simulink library "SUB_ECU_L4_MABX_HW_Interface"  (R2018a)
settings: Solver=VariableStepAuto  StartTime=0.0  StopTime=10.0  RelTol=1e-3
PostLoadFcn:
  | , if any(exist('dsrtsu_mdlpostloadfcn', 'file') == [2, 3, 6]), try dsrtsu_mdlpostloadfcn('Execute', bdroot); catch fprintf('Error in PostLoadFcn (dsrtsu_mdlpostloadfcn) for model "%s":\n %s\n', bdroot, lasterr); end, end,
undefined symbols (not defined in the file or in its folder): CANR_PROPB_REAX_3_13_CHANNEL_APV, CANR_PROPB_REAX_4_13_CHANNEL_APV, CANR_PROPB_XPR_1_50_CHANNEL_APV, ENUM_CAN_RX_T, ENUM_CAN_TX_T, ENUM_REAX_OPERATION_MODE_T, ENUM_SIGNAL_HEALTH_T, ENUM_XBR_CONTROL_MODE_T, ENUM_XBR_EBI_MODE_T, ENUM_XBR_PASS_THROUGH_ACTIVE_T, ENUM_XBR_PRIORITY_T, ENUM_XPR_INHIBIT_PARK_MANUAL_T, ENUM_XPR_INHIBIT_UNPARK_MANUAL_T, ENUM_XPR_PARK_MANUAL_T, ENUM_XPR_UNPARK_MANUAL_T, PROPB_REAX_1_E4_DES_POS_SIG_SRC_APV, PROPB_REAX_1_E4_DESIRED_OPMODE_APV, PROPB_REAX_1_E4_DESIRED_POSITION_APV, ptc_matlab_lib
libraries: PTC_MBDS_LIB x264, rtican x172, EmE_MBD_Blockset x39, simulink x34, $bdroot x16, rti1401lib_dio_type4 x8, simulink_need_slupdate x7, dsa_tcpip_lib x4, rti1401lib_adc_type4 x3, rtmapslib x3, rtitasklib x3
(part 48 of 51)

== system SUB_ECU_L4_MABX_HW_Interface/CAN_Out_PTC_1571/CAN_TX_100ms/Encode_PropB_XPR_FC/Encode_PropB_XPR_FC_checksum ==
  byte1 : Inport  OutDataTypeStr=uint8
  byte2 : Inport  Port=2  OutDataTypeStr=uint8
  byte3 : Inport  Port=3
  byte4 : Inport  Port=4
  byte5 : Inport  Port=5
  byte6 : Inport  Port=6
  byte7 : Inport  Port=7
  Counter : Inport  Port=8
  MessageID : Inport  Port=9
  AND1 : PTC_MBDS_LIB/MBDS Standard Library/Basic Operations/Logic and Bit Operations/AND  BitwiseMode=on  Inputs=1  UseBitMask=on  BitMask='0F'  OutDataTypeStr=uint8  PTC_MBDS_BlockVersion=5.41  PTC_BlockType=PTC_MBDS_AND
      settings: AttributesFormatString=bitwise  SourceProductName=PACCAR Technical Center MBDS Library
  AND10 : PTC_MBDS_LIB/MBDS Standard Library/Basic Operations/Logic and Bit Operations/AND  BitwiseMode=on  Inputs=1  UseBitMask=on  BitMask='0F'  OutDataTypeStr=uint8  PTC_MBDS_BlockVersion=5.41  PTC_BlockType=PTC_MBDS_AND
      settings: AttributesFormatString=bitwise  SourceProductName=PACCAR Technical Center MBDS Library
  AND5 : PTC_MBDS_LIB/MBDS Standard Library/Basic Operations/Logic and Bit Operations/AND  BitwiseMode=on  Inputs=1  UseBitMask=on  BitMask='000000FF'  OutDataTypeStr=uint8  PTC_MBDS_BlockVersion=5.41  PTC_BlockType=PTC_MBDS_AND
      settings: AttributesFormatString=bitwise  SourceProductName=PACCAR Technical Center MBDS Library
  AND6 : PTC_MBDS_LIB/MBDS Standard Library/Basic Operations/Logic and Bit Operations/AND  BitwiseMode=on  Inputs=1  UseBitMask=on  BitMask='0000FF00'  OutDataTypeStr=uint16  PTC_MBDS_BlockVersion=5.41  PTC_BlockType=PTC_MBDS_AND
      settings: AttributesFormatString=bitwise  SourceProductName=PACCAR Technical Center MBDS Library
  AND7 : PTC_MBDS_LIB/MBDS Standard Library/Basic Operations/Logic and Bit Operations/AND  BitwiseMode=on  Inputs=1  UseBitMask=on  BitMask='00FF0000'  OutDataTypeStr=uint32  PTC_MBDS_BlockVersion=5.41  PTC_BlockType=PTC_MBDS_AND
      settings: AttributesFormatString=bitwise  SourceProductName=PACCAR Technical Center MBDS Library
  AND8 : PTC_MBDS_LIB/MBDS Standard Library/Basic Operations/Logic and Bit Operations/AND  BitwiseMode=on  Inputs=1  UseBitMask=on  BitMask='FF000000'  OutDataTypeStr=uint32  PTC_MBDS_BlockVersion=5.41  PTC_BlockType=PTC_MBDS_AND
      settings: AttributesFormatString=bitwise  SourceProductName=PACCAR Technical Center MBDS Library
  Add : Sum  Inputs=++++++++++++  OutDataTypeStr=uint8  InputSameDT=on
      settings: AttributesFormatString=Saturate: %<SaturateOnIntegerOverflow>
  Add1 : Sum  OutDataTypeStr=uint8  InputSameDT=on
      settings: AttributesFormatString=Saturate: %<SaturateOnIntegerOverflow>
  Data Type Conversion10 : DataTypeConversion  OutDataTypeStr=uint8  SaturateOnIntegerOverflow=on
  Data Type Conversion11 : DataTypeConversion  OutDataTypeStr=uint8  SaturateOnIntegerOverflow=on
  Data Type Conversion13 : DataTypeConversion  OutMin=0  OutMax=15  OutDataTypeStr=uint8  SaturateOnIntegerOverflow=on
  Data Type Conversion8 : DataTypeConversion  OutDataTypeStr=uint32  SaturateOnIntegerOverflow=on
  Data Type Conversion9 : DataTypeConversion  OutDataTypeStr=uint8  SaturateOnIntegerOverflow=on
  Shift_Arithmetic 3 : ArithShift  BitShiftNumber=8
  Shift_Arithmetic 4 : ArithShift  BitShiftNumber=16
  Shift_Arithmetic 5 : ArithShift  BitShiftNumber=24
  Shift_Arithmetic 7 : ArithShift  BitShiftNumber=4
  Data : Outport
  wires:
  MessageID/1 -> Data Type Conversion8/1
  Data Type Conversion8/1 -> AND8/1, AND7/1, AND6/1, AND5/1
  AND5/1 -> Add/8  "MessageIDLowByte"
  AND6/1 -> Shift_Arithmetic 3/1
  Shift_Arithmetic 3/1 -> Data Type Conversion9/1
  Data Type Conversion9/1 -> Add/9  "MessageIDMidLowByte"
  AND7/1 -> Shift_Arithmetic 4/1
  Shift_Arithmetic 4/1 -> Data Type Conversion10/1
  Data Type Conversion10/1 -> Add/10  "MessageIDMidHighByte"
  AND8/1 -> Shift_Arithmetic 5/1
  Shift_Arithmetic 5/1 -> Data Type Conversion11/1
  Data Type Conversion11/1 -> Add/11  "MessageIDHighByte"
  AND10/1 -> Add/12
  AND1/1 -> Data/1
  Counter/1 -> Data Type Conversion13/1
  Data Type Conversion13/1 -> AND10/1
  byte1/1 -> Add/1
  byte2/1 -> Add/2
  byte3/1 -> Add/3
  byte4/1 -> Add/4
  byte5/1 -> Add/5
  byte6/1 -> Add/6
  byte7/1 -> Add/7
  Add/1 -> Add1/2, Shift_Arithmetic 7/1  "Checksum"
  Shift_Arithmetic 7/1 -> Add1/1
  Add1/1 -> AND1/1

== system SUB_ECU_L4_MABX_HW_Interface/CAN_Out_PTC_1571/CAN_TX_100ms/Encode_PropB_XPR_FC/MessageID ==
  note: 0x18FF04FC
  Data Type Conversion{,1..5} (6 alike) : DataTypeConversion  OutDataTypeStr=uint32  SaturateOnIntegerOverflow=on
  DataPage : Constant  Value=boolean(0)
  ExtendedDataPage : Constant  Value=boolean(0)
  OR : PTC_MBDS_LIB/MBDS Standard Library/Basic Operations/Logic and Bit Operations/OR  BitwiseMode=on  Inputs=6  UseBitMask=off  BitMask='A7'  OutDataTypeStr=Inherit: Inherit via back propagation  PTC_MBDS_BlockVersion=5.41  PTC_BlockType=PTC_MBDS_OR
      settings: AttributesFormatString=bitwise  SourceProductName=PACCAR Technical Center MBDS Library
  PDUFormat : Constant  Value=uint8(hex2dec('FF'))
  PDUSpecific : Constant  Value=uint8(hex2dec('04'))
  Priority : Constant  Value=uint8(6)
  "Shift_Arithmetic " : ArithShift  BitShiftNumber=-26
  Shift_Arithmetic 1 : ArithShift  BitShiftNumber=-25
  Shift_Arithmetic 2 : ArithShift  BitShiftNumber=-24
  Shift_Arithmetic 3 : ArithShift  BitShiftNumber=-16
  Shift_Arithmetic 4 : ArithShift  BitShiftNumber=-8
  SourceAddress : Constant  Value=uint8(hex2dec('FC'))
  MessageID : Outport
  wires:
  Shift_Arithmetic 3/1 -> OR/4
  Shift_Arithmetic 4/1 -> OR/5
  Shift_Arithmetic 2/1 -> OR/3
  Shift_Arithmetic 1/1 -> OR/2
  "Shift_Arithmetic "/1 -> OR/1
  Data Type Conversion5/1 -> OR/6
  SourceAddress/1 -> Data Type Conversion5/1
  Data Type Conversion4/1 -> Shift_Arithmetic 4/1
  PDUSpecific/1 -> Data Type Conversion4/1
  Data Type Conversion3/1 -> Shift_Arithmetic 3/1
  PDUFormat/1 -> Data Type Conversion3/1
  Data Type Conversion2/1 -> Shift_Arithmetic 2/1
  DataPage/1 -> Data Type Conversion2/1
  Data Type Conversion1/1 -> Shift_Arithmetic 1/1
  ExtendedDataPage/1 -> Data Type Conversion1/1
  Data Type Conversion/1 -> "Shift_Arithmetic "/1
  Priority/1 -> Data Type Conversion/1
  OR/1 -> MessageID/1

== system SUB_ECU_L4_MABX_HW_Interface/CAN_Out_PTC_1571/CAN_TX_100ms/Encode_PropB_XPR_FC/Rolling_15_counter ==
  Enable : EnablePort  ZeroCross=off
      settings: AttributesFormatString=States when enabling: %<StatesWhenEnabling>
  Increment Real World1 : simulink/Additional Math & Discrete/Additional Math: Increment - Decrement/Increment Real World  DisableCoverage=on
      settings: SourceProductName=Simulink  SourceProductBaseCode=SL
  Unit_Delay : UnitDelay  SampleTime=-1
      settings: AttributesFormatString=IC: %<vinit>
  Wrap To Zero1 : simulink/Discontinuities/Wrap To Zero  DisableCoverage=on  Threshold=15
      settings: SourceProductName=Simulink  SourceProductBaseCode=SL
  Rolling_15_counter : Outport  InitialOutput=15
      settings: AttributesFormatString=IC: %<InitialOutput>\nDisabled Value: %<OutputWhenDisabled>\n
  wires:
  Unit_Delay/1 -> Rolling_15_counter/1, Increment Real World1/1
  Wrap To Zero1/1 -> Unit_Delay/1
  Increment Real World1/1 -> Wrap To Zero1/1

== system SUB_ECU_L4_MABX_HW_Interface/CAN_Out_PTC_1571/CAN_TX_100ms/POSRapidUpdate/TX ==
  Enable : Inport
  Data : Inport  Port=2
  Bus Selector : BusSelector  OutputSignals=INPUTS.CAN.PosRapidUpdate.Latitude_,INPUTS.CAN.PosRapidUpdate.Longitude_
  Data Type Conversion : DataTypeConversion  OutDataTypeStr=double
  Data Type Conversion1 : DataTypeConversion  OutDataTypeStr=double
  Std_PosRapidUpdate_01 : rtican/RTICAN Transmit (TX)   Reserved1=[]  Reserved2=[]  Reserved3=[]  Reserved4=[]  SfcnMessage=[]  Msg_Struct=[]  BoardTypeNo=[]  BoardNo=[]  ChannelNo=[]  Parameters=[]  DialogFcn=[]  UnitName=[]  Revision=[]  UnitValues=[]  DSProperties=struct('RTI',struct('Version',uint32(5),'BlockType',struct('isSLSource',uint8(1),'isSLSink',uint8(1),'isHWSource',uint8(0),'isHWSink',uint8(0),'isSetup',uint8(0),'isInline',uint8(1),'isNonInline',uint8(0),'isInterrupt',uint8(0),'isChannelwise',uint8(0)),'IOBoardType','RTICAN','UnitType','MESSAGE','Identifier','TX','DialogType','MSVC','BlockSet','RTICAN','SlaveProcessor','CAN'))  RTIBlockInterface=struct('InputPortsWidth',int32([1 1]),'InputPortsActive',[1 1],'InputPortsName',{{'Latitude_','Longitude_'}},'InputPortsDataType',{{'SS_DOUBLE','SS_DOUBLE'}},'OutputPortsWidth',int32([1 1 1 1]),'OutputPortsActive',[1 1 1 1],'OutputPortsName',{{['TX status'],['TX time'],['TX delta time'],['TX delay time']}},'DialogFcn','rtican_message_interface_gui','BlockDisplay',{{'','center'}},'IconTransparency','on','InitLevel',3,'BlockName',struct('Token',{{'Std_PosRapidUpdate_01'}}),'SampleTime',{{-1}},'TriggerPort',{{'none'}},'EnablePort',{{'yes'}})  RTIBlockParameters=struct('BoardTypeNo',{{1,'OFF',[]}},'BoardNo',{{3,'ON',[1 16]}},'ChannelNo',{{2,'ON',[1 2]}},'Parameters',{{struct('DataFileSupport',struct('DataFileSelectedMaster',1,'DataFileSelectedLocal',0,'DataFileName','c:\data\svn\truck1571\dbc\mabx_can6.dbc|c:\data\svn\candb\mabx_can4_chrisbalton.dbc|','DataFileDate',{{{['12-Oct-2017 12:26:19']},{''}}},'SelectedFile',['<no file selected>']),'Options',struct('StatusSelected',1,'TimeSelected',1,'DeltaTimeSelected',1,'DelayTimeSelected',1,'DelayTimeTXCommandSelected',0,'EncodeSetUnusedBitsToOne',1,'EnableMsgLoopback',0,'TriggerPort',struct('Selected',0,'TriggerType',0),'EnablePortSelected',1,'SignalOnPortnameSelected',1,'UserCoding',struct('Selected',0,'InterfaceFile','UserEncodingFile','FcnName','UserEncodeFcn','InportSelected',0,'InportWidth',1,'OutportSelected',0,'OutportWidth',1),'TerminationMsg',struct('Selected',0,'Byte0_7','0'),'InitialMsg',struct('Selected',0,'Byte0_7','0')),'Message',struct('MsgOnBlocknameSelected',1,'MsgName','Std_PosRapidUpdate_01','MsgIdFormat',0,'MsgId',3,'MsgLength',8,'NumSignals',2,'SampleTime',-1,'StartTime',struct('Selected',0,'Value',0),'AutoRepeatTime',struct('Selected',0,'Value',0.1),'Timeout',struct('Selected',0,'Value',0.1),'DelayTime',struct('Selected',0,'Value',0.1),'Signal',struct('SgnName',{'Latitude_','Longitude_'},'SgnStartBit',{0,32},'SgnLength',{32,32},'SgnType',{0,0},'ModeValue',{-1,-1},'DataType',{1,1},'ByteLayout',{0,0},'Factor',{1e-7,1e-7},'Offset',{0,0},'SgnComment',{{''},{''}},'SgnUnit',{'deg','deg'},'Min',{-90,-180},'Max',{90,180},'SLDataType',{'SS_DOUBLE','SS_DOUBLE'}),'MsgIdNumFormat',0,'MsgComment',{{['This PGN provides latitude and longitude referenced to WGS84.Being defined as single frame Msg,as ']}}),'Version',1.2,'general',struct('isFromLib',0)),'OFF',[]}},'GroupId',{{struct('Group',{{'RTICAN'}},'No',6,'Behavior',{{'NAMECHANGE'}},'BlockType',{{'SINK'}},'NameChangeFlag',0),'OFF',[]}},'SFcnRTICANMessage',{{struct('MsgType','TX','SFcnPortType','Scalar','MsgName','Std_PosRapidUpdate_01','MsgIdFormat','STD','MsgId',3,'MsgLength',8,'NumSignals',2,'SampleTime',-1,'StartTime',struct('Selected','no','Value',0),'AutoRepeatTime',struct('Selected','no','Value',0.1),'Timeout',struct('Selected','no','Value',0.1),'Signal',struct('SgnName',{'Latitude_','Longitude_'},'SgnStartBit',{0,32},'SgnLength',{32,32},'SgnType',{'standard','standard'},'ModeValue',{-1,-1},'DataType',{['signed int'],['signed int']},'ByteLayout',{['little endian'],['little endian']},'Factor',{1e-7,1e-7},'Offset',{0,0},'SLDataType',{'SS_DOUBLE','SS_DOUBLE'}),'StatusSelected','yes','TimeSelected','yes','DeltaTimeSelected','yes','DelayTimeSelected','yes','DelayTimeTXCommandSelected','no','EncodeSetUnusedBitsToOne','yes','EnableMsgLoopback','no','TriggerPort',struct('Selected','no','TriggerType',0),'EnablePortSelected','yes','UserCoding',struct('Selected','no','InterfaceFile','UserEncodingFile','FcnName','UserEncodeFcn','InportSelected','no','InportWidth',1,'OutportSelected','no','OutportWidth',1),'TerminationMsg',struct('Selected','no','Byte0','0x00','Byte1','0x00','Byte2','0x00','Byte3','0x00','Byte4','0x00','Byte5','0x00','Byte6','0x00','Byte7','0x00'),'InitialMsg',struct('Selected','no','Byte0','0x00','Byte1','0x00','Byte2','0x00','Byte3','0x00','Byte4','0x00','Byte5','0x00','Byte6','0x00','Byte7','0x00'),'BoardType','DS1','BoardNo',3,'ControllerNo',2),'OFF',[]}},'TLCFileName',{{'rtican_tx_message','OFF',[]}})  RTISFcnParameters=struct('SFcnRTICANMessage','struct','TLCFileName','char')  RTIBlockParaDefault=struct('BoardTypeNo',4302,'BoardNo',1,'ChannelNo',1,'Parameters',struct('DataFileSupport',struct('DataFileSelectedMaster',0,'DataFileSelectedLocal',0,'DataFileName','','DataFileDate','','SelectedFile',['<no file selected>']),'Options',struct('StatusSelected',1,'TimeSelected',1,'DeltaTimeSelected',1,'DelayTimeSelected',1,'DelayTimeTXCommandSelected',0,'EncodeSetUnusedBitsToOne',0,'EnableMsgLoopback',0,'TriggerPort',struct('Selected',0,'TriggerType','rising'),'EnablePortSelected',0,'SignalOnPortnameSelected',1,'UserCoding',struct('Selected',0,'InterfaceFile','UserEncodingFile','FcnName','UserEncodeFcn','InportSelected',0,'InportWidth',1,'OutportSelected',0,'OutportWidth',1),'TerminationMsg',struct('Selected',0,'Byte0_7','0'),'InitialMsg',struct('Selected',0,'Byte0_7','0')),'Message',struct('MsgOnBlocknameSelected',0,'MsgName',['TX Message'],'MsgIdFormat',0,'MsgId',100,'MsgLength',8,'NumSignals',1,'SampleTime',-1,'StartTime',struct('Selected',0,'Value',0),'AutoRepeatTime',struct('Selected',0,'Value',0.1),'Timeout',struct('Selected',0,'Value',0.1),'DelayTime',struct('Selected',0,'Value',0.1),'Signal',struct('SgnName',['TX signal'],'SgnStartBit',0,'SgnLength',8,'SgnType',0,'ModeValue',-1,'DataType',0,'SLDataType','SS_DOUBLE','ByteLayout',0,'Factor',1,'Offset',0,'Min',0,'Max',255,'SgnComment',{{}},'SgnUnit',''),'MsgIdNumFormat',0,'MsgComment',{{''}}),'Version',1.2,'general',struct('isFromLib',1)),'GroupId',struct('Group',{{'RTICAN'}},'No',1,'Behavior',{{'NAMECHANGE'}},'BlockType',{{'SINK'}},'NameChangeFlag',0),'SFcnRTICANMessage',struct('MsgType','TX','MsgName',['TX Message'],'MsgIdFormat','STD','MsgId',100,'MsgLength',2,'NumSignals',1,'SampleTime',-1,'StartTime',struct('Selected','no','Value',0),'AutoRepeatTime',struct('Selected','no','Value',0.1),'Timeout',struct('Selected','no','Value',0.1),'DelayTime',struct('Selected','no','Value',0.1),'Signal',struct('SgnName',['TX signal'],'SgnStartBit',0,'SgnLength',8,'SgnType','standard','ModeValue',-1,'DataType',['unsigned int'],'ByteLayout',['little endian'],'SLDataType','SS_DOUBLE','Factor',1,'Offset',0),'StatusSelected','yes','TimeSelected','yes','DeltaTimeSelected','yes','DelayTimeSelected','yes','EnablePortSelected','no','EnableMsgLoopback','no','DelayTimeTXCommandSelected','no','EncodeSetUnusedBitsToOne','no','UserCoding',struct('Selected','no','InterfaceFile','UserDecodingFile','FcnName','UserDecodeFcn','InportSelected','no','InportWidth',1,'OutportSelected','no','OutportWidth',1),'TerminationMsg',struct('Selected','no','Byte0','0x00','Byte1','0x00','Byte2','0x00','Byte3','0x00','Byte4','0x00','Byte5','0x00','Byte6','0x00','Byte7','0x00'),'InitialMsg',struct('Selected','no','Byte0','0x00','Byte1','0x00','Byte2','0x00','Byte3','0x00','Byte4','0x00','Byte5','0x00','Byte6','0x00','Byte7','0x00'),'TriggerPort',struct('Selected','no','TriggerType','rising'),'BoardType','DS4302','BoardNo',1,'ControllerNo',1,'SFcnPortType','Scalar'),'TLCFileName','rtican_tx_message')
      settings: AttributesFormatString=Group Id: RTICAN6\n  SourceProductName=dSPACE RTI CAN Blockset
  Terminator{,1..3} (4 alike) : Terminator
      settings: InitFcn=|
      | try
      |    MBDS_BlockCallback('Update', gcb);
      | end
  wires:
  Data Type Conversion1/1 -> Std_PosRapidUpdate_01/2
  Data Type Conversion/1 -> Std_PosRapidUpdate_01/1
  Enable/1 -> Std_PosRapidUpdate_01/Enable
  Std_PosRapidUpdate_01/2 -> Terminator1/1
  Std_PosRapidUpdate_01/4 -> Terminator3/1
  Std_PosRapidUpdate_01/3 -> Terminator2/1
  Std_PosRapidUpdate_01/1 -> Terminator/1
  Data/1 -> Bus Selector/1
  Bus Selector/1 -> Data Type Conversion/1  "<Latitude_>"
  Bus Selector/2 -> Data Type Conversion1/1  "<Longitude_>"

== system SUB_ECU_L4_MABX_HW_Interface/CAN_Out_PTC_1571/CAN_TX_10ms/CAN_TX_ACCS_E4/TX_CAN4 ==
  note: THIS MESSAGE EXISTS FOR CANALYZER DEBUGGING PURPOSES
      | ONLY AND HAS NO CONTROLLERS EXPECTING TO RECEIVE IT ON ANY CAN BUS
  Enable : Inport
  Data : Inport  Port=2
  ACCS : rtican/RTICAN Transmit (TX)   Reserved1=[]  Reserved2=[]  Reserved3=[]  Reserved4=[]  SfcnMessage=[]  Msg_Struct=[]  BoardTypeNo=[]  BoardNo=[]  ChannelNo=[]  Parameters=[]  DialogFcn=[]  UnitName=[]  Revision=[]  UnitValues=[]  DSProperties=struct('RTI',struct('Version',uint32(5),'BlockType',struct('isSLSource',uint8(1),'isSLSink',uint8(1),'isHWSource',uint8(0),'isHWSink',uint8(0),'isSetup',uint8(0),'isInline',uint8(1),'isNonInline',uint8(0),'isInterrupt',uint8(0),'isChannelwise',uint8(0)),'IOBoardType','RTICAN','UnitType','MESSAGE','Identifier','TX','DialogType','MSVC','BlockSet','RTICAN','SlaveProcessor','CAN'))  RTIBlockInterface=struct('InputPortsWidth',int32(1),'InputPortsActive',1,'InputPortsName',{{'LongitudinalAccelerationExRange'}},'InputPortsDataType',{{'SS_DOUBLE'}},'OutputPortsWidth',int32([1 1 1 1]),'OutputPortsActive',[1 1 1 1],'OutputPortsName',{{['TX status'],['TX time'],['TX delta time'],['TX delay time']}},'DialogFcn','rtican_message_interface_gui','BlockDisplay',{{'','center'}},'IconTransparency','on','InitLevel',3,'BlockName',struct('Token',{{'ACCS'}}),'SampleTime',{{-1}},'TriggerPort',{{'none'}},'EnablePort',{{'yes'}})  RTIBlockParameters="struct('BoardTypeNo',{{1,'OFF',[]}},'BoardNo',{{2,'ON',[1 16]}},'ChannelNo',{{2,'ON',[1 2]}},'Parameters',{{struct('DataFileSupport',struct('DataFileSelectedMaster',1,'DataFileSelectedLocal',0,'DataFileName',['c:\\data\\svn\\truck1571\\dbc\\mabx_can4.dbc|c:\\data\\svn\\svn\\powertrainsys\\trunk\\src\\projects_rcp\\my2017_rcp\\dbc files\\j1939.dbc|'],'DataFileDate',{{{['10-Feb-2017 15:17:28']},{['24-Aug-2017 12:01:59']}}},'SelectedFile',['<no file selected>']),'Options',struct('StatusSelected',1,'TimeSelected',1,'DeltaTimeSelected',1,'DelayTimeSelected',1,'DelayTimeTXCommandSelected',0,'EncodeSetUnusedBitsToOne',1,'EnableMsgLoopback',0,'TriggerPort',struct('Selected',0,'TriggerType',0),'EnablePortSelected',1,'SignalOnPortnameSelected',1,'UserCoding',struct('Selected',0,'InterfaceFile','UserEncodingFile','FcnName','UserEncodeFcn','InportSelected',0,'InportWidth',1,'OutportSelected',0,'OutportWidth',1),'TerminationMsg',struct('Selected',0,'Byte0_7','0'),'InitialMsg',struct('Selected',0,'Byte0_7','0')),'Message',struct('MsgOnBlocknameSelected',1,'MsgName','ACCS','MsgIdFormat',1,'MsgId',418393572,'MsgLength',8,'NumSignals',1,'SampleTime',-1,'StartTime',struct('Selected',0,'Value',0),'AutoRepeatTime',struct('Selected',0,'Value',0.1),'Timeout',struct('Selected',0,'Value',0.1),'DelayTime',struct('Selected',0,'Value',0.1),'Signal',struct('SgnName','LongitudinalAccelerationExRange','SgnStartBit',16,'SgnLength',16,'SgnType',0,'ModeValue',-1,'DataType',0,'ByteLayout',0,'Factor',0.01,'Offset',-320,'SgnComment',{{['Indicates longitudinal acceleration of the vehicle (the component of vehicle acceleration vector along the X-axis).  A positive longitudinal acceleration signal results when the vehicle speed increases in the forward direction.  Longitudinal ...']}},'SgnUnit','m/s²','Min',-320,'Max',322.55,'SLDataType','SS_DOUBLE'),'MsgIdNumFormat',1,'MsgComment',{{['Acceleration Sensor' char(10) 'The acceleration sensor message shall provide a measurement of the vehicle''s ']}}),'Version',1.2,'general',struct('isFromLib',0)),'OFF',[]}},'GroupId',{{struct('Group',{{'RTICAN'}},'No',4,'Behavior',{{'NAMECHANGE'}},'BlockType',{{'SINK'}},'NameChangeFlag',0),'OFF',[]}},'SFcnRTICANMessage',{{struct('MsgType','TX','SFcnPortType','Scalar','MsgName','ACCS','MsgIdFormat','XTD','MsgId',418393572,'MsgLength',8,'NumSignals',1,'SampleTime',-1,'StartTime',struct('Selected','no','Value',0),'AutoRepeatTime',struct('Selected','no','Value',0.1),'Timeout',struct('Selected','no','Value',0.1),'Signal',struct('SgnName','LongitudinalAccelerationExRange','SgnStartBit',16,'SgnLength',16,'SgnType','standard','ModeValue',-1,'DataType',['unsigned int'],'ByteLayout',['little endian'],'Factor',0.01,'Offset',-320,'SLDataType','SS_DOUBLE'),'StatusSelected','yes','TimeSelected','yes','DeltaTimeSelected','yes','DelayTimeSelected','yes','DelayTimeTXCommandSelected','no','EncodeSetUnusedBitsToOne','yes','EnableMsgLoopback','no','TriggerPort',struct('Selected','no','TriggerType',0),'EnablePortSelected','yes','UserCoding',struct('Selected','no','InterfaceFile','UserEncodingFile','FcnName','UserEncodeFcn','InportSelected','no','InportWidth',1,'OutportSelected','no','OutportWidth',1),'TerminationMsg',struct('Selected','no','Byte0','0x00','Byte1','0x00','Byte2','0x00','Byte3','0x00','Byte4','0x00','Byte5','0x00','Byte6','0x00','Byte7','0x00'),'InitialMsg',struct('Selected','no','Byte0','0x00','Byte1','0x00','Byte2','0x00','Byte3','0x00','Byte4','0x00','Byte5','0x00','Byte6','0x00','Byte7','0x00'),'BoardType','DS1','BoardNo',2,'ControllerNo',2),'OFF',[]}},'TLCFileName',{{'rtican_tx_message','OFF',[]}})"  RTISFcnParameters=struct('SFcnRTICANMessage','struct','TLCFileName','char')  RTIBlockParaDefault=struct('BoardTypeNo',4302,'BoardNo',1,'ChannelNo',1,'Parameters',struct('DataFileSupport',struct('DataFileSelectedMaster',0,'DataFileSelectedLocal',0,'DataFileName','','DataFileDate','','SelectedFile',['<no file selected>']),'Options',struct('StatusSelected',1,'TimeSelected',1,'DeltaTimeSelected',1,'DelayTimeSelected',1,'DelayTimeTXCommandSelected',0,'EncodeSetUnusedBitsToOne',0,'EnableMsgLoopback',0,'TriggerPort',struct('Selected',0,'TriggerType','rising'),'EnablePortSelected',0,'SignalOnPortnameSelected',1,'UserCoding',struct('Selected',0,'InterfaceFile','UserEncodingFile','FcnName','UserEncodeFcn','InportSelected',0,'InportWidth',1,'OutportSelected',0,'OutportWidth',1),'TerminationMsg',struct('Selected',0,'Byte0_7','0'),'InitialMsg',struct('Selected',0,'Byte0_7','0')),'Message',struct('MsgOnBlocknameSelected',0,'MsgName',['TX Message'],'MsgIdFormat',0,'MsgId',100,'MsgLength',8,'NumSignals',1,'SampleTime',-1,'StartTime',struct('Selected',0,'Value',0),'AutoRepeatTime',struct('Selected',0,'Value',0.1),'Timeout',struct('Selected',0,'Value',0.1),'DelayTime',struct('Selected',0,'Value',0.1),'Signal',struct('SgnName',['TX signal'],'SgnStartBit',0,'SgnLength',8,'SgnType',0,'ModeValue',-1,'DataType',0,'SLDataType','SS_DOUBLE','ByteLayout',0,'Factor',1,'Offset',0,'Min',0,'Max',255,'SgnComment',{{}},'SgnUnit',''),'MsgIdNumFormat',0,'MsgComment',{{''}}),'Version',1.2,'general',struct('isFromLib',1)),'GroupId',struct('Group',{{'RTICAN'}},'No',1,'Behavior',{{'NAMECHANGE'}},'BlockType',{{'SINK'}},'NameChangeFlag',0),'SFcnRTICANMessage',struct('MsgType','TX','MsgName',['TX Message'],'MsgIdFormat','STD','MsgId',100,'MsgLength',2,'NumSignals',1,'SampleTime',-1,'StartTime',struct('Selected','no','Value',0),'AutoRepeatTime',struct('Selected','no','Value',0.1),'Timeout',struct('Selected','no','Value',0.1),'DelayTime',struct('Selected','no','Value',0.1),'Signal',struct('SgnName',['TX signal'],'SgnStartBit',0,'SgnLength',8,'SgnType','standard','ModeValue',-1,'DataType',['unsigned int'],'ByteLayout',['little endian'],'SLDataType','SS_DOUBLE','Factor',1,'Offset',0),'StatusSelected','yes','TimeSelected','yes','DeltaTimeSelected','yes','DelayTimeSelected','yes','EnablePortSelected','no','EnableMsgLoopback','no','DelayTimeTXCommandSelected','no','EncodeSetUnusedBitsToOne','no','UserCoding',struct('Selected','no','InterfaceFile','UserDecodingFile','FcnName','UserDecodeFcn','InportSelected','no','InportWidth',1,'OutportSelected','no','OutportWidth',1),'TerminationMsg',struct('Selected','no','Byte0','0x00','Byte1','0x00','Byte2','0x00','Byte3','0x00','Byte4','0x00','Byte5','0x00','Byte6','0x00','Byte7','0x00'),'InitialMsg',struct('Selected','no','Byte0','0x00','Byte1','0x00','Byte2','0x00','Byte3','0x00','Byte4','0x00','Byte5','0x00','Byte6','0x00','Byte7','0x00'),'TriggerPort',struct('Selected','no','TriggerType','rising'),'BoardType','DS4302','BoardNo',1,'ControllerNo',1,'SFcnPortType','Scalar'),'TLCFileName','rtican_tx_message')
      settings: AttributesFormatString=Group Id: RTICAN4\n  SourceProductName=dSPACE RTI CAN Blockset
  Bus Selector : BusSelector  OutputSignals=10msTask.BrakeCtrl.Accel_rate_ms2
  Data Type Conversion4 : DataTypeConversion  OutDataTypeStr=double  SaturateOnIntegerOverflow=on
  Terminator{,1..3} (4 alike) : Terminator
      settings: InitFcn=|
      | try
      |    MBDS_BlockCallback('Update', gcb);
      | end
  wires:
  Data Type Conversion4/1 -> ACCS/1
  ACCS/2 -> Terminator1/1
  ACCS/4 -> Terminator3/1
  ACCS/3 -> Terminator2/1
  ACCS/1 -> Terminator/1
  Enable/1 -> ACCS/Enable
  Data/1 -> Bus Selector/1
  Bus Selector/1 -> Data Type Conversion4/1  "<Accel_rate_ms2>"

== system SUB_ECU_L4_MABX_HW_Interface/CAN_Out_PTC_1571/CAN_TX_10ms/CAN_TX_EEC1_00/TX_CAN4 ==
  Enable : Inport
  Data : Inport  Port=2
  Bus Selector : BusSelector  OutputSignals=INPUTS.CAN.EEC1_00.EngTorqueMode,INPUTS.CAN.EEC1_00.ActlEngPrcntTrqueHighResolution,INPUTS.CAN.EEC1_00.DriversDemandEngPercentTorque,INPUTS.CAN.EEC1_00.ActualEngPercentTorque,INPUTS.CAN.EEC1_00.EngSpeed,INPUTS.CAN.EEC1_00.SrcAddrssOfCtrllngDvcFrEngCntrl,INPUTS.CAN.EEC1_00.EngStarterMode,INPUTS.CAN.EEC1_00.EngDemandPercentTorque
  Data Type Conversion{1..8} (8 alike) : DataTypeConversion  OutDataTypeStr=double  SaturateOnIntegerOverflow=on
  EEC1_00 : rtican/RTICAN Transmit (TX)   Reserved1=[]  Reserved2=[]  Reserved3=[]  Reserved4=[]  SfcnMessage=[]  Msg_Struct=[]  BoardTypeNo=[]  BoardNo=[]  ChannelNo=[]  Parameters=[]  DialogFcn=[]  UnitName=[]  Revision=[]  UnitValues=[]  DSProperties=struct('RTI',struct('Version',uint32(5),'BlockType',struct('isSLSource',uint8(1),'isSLSink',uint8(1),'isHWSource',uint8(0),'isHWSink',uint8(0),'isSetup',uint8(0),'isInline',uint8(1),'isNonInline',uint8(0),'isInterrupt',uint8(0),'isChannelwise',uint8(0)),'IOBoardType','RTICAN','UnitType','MESSAGE','Identifier','TX','DialogType','MSVC','BlockSet','RTICAN','SlaveProcessor','CAN'))  RTIBlockInterface=struct('InputPortsWidth',int32([1 1 1 1 1 1 1 1]),'InputPortsActive',[1 1 1 1 1 1 1 1],'InputPortsName',{{'SPN899_EngineTorqueMode','SPN4154_ActEngPercTorqueFrac','SPN512_DrvrDemEngPercTrq','SPN513_ActEngPercTorque','SPN190_EngineSpeed','SPN1483_SAOfCtrlDevForEngineCtrl','SPN1675_EngineStarterMode','SPN2432_EngDemPercTrq'}},'InputPortsDataType',{{'SS_DOUBLE','SS_DOUBLE','SS_DOUBLE','SS_DOUBLE','SS_DOUBLE','SS_DOUBLE','SS_DOUBLE','SS_DOUBLE'}},'OutputPortsWidth',int32([1 1 1 1]),'OutputPortsActive',[1 1 1 1],'OutputPortsName',{{['TX status'],['TX time'],['TX delta time'],['TX delay time']}},'DialogFcn','rtican_message_interface_gui','BlockDisplay',{{'','center'}},'IconTransparency','on','InitLevel',3,'BlockName',struct('Token',{{'EEC1_00'}}),'SampleTime',{{-1}},'TriggerPort',{{'none'}},'EnablePort',{{'yes'}})  RTIBlockParameters=struct('BoardTypeNo',{{1,'OFF',[]}},'BoardNo',{{2,'ON',[1 16]}},'ChannelNo',{{2,'ON',[1 2]}},'Parameters',{{struct('DataFileSupport',struct('DataFileSelectedMaster',1,'DataFileSelectedLocal',0,'DataFileName',['c:\data\svn\truck1571\dbc\mabx_can4.dbc|c:\data\svn\svn\powertrainsys\trunk\src\projects_rcp\my2017_rcp\dbc files\j1939.dbc|'],'DataFileDate',{{{['16-Jan-2018 13:46:56']}}},'SelectedFile',['<no file selected>']),'Options',struct('StatusSelected',1,'TimeSelected',1,'DeltaTimeSelected',1,'DelayTimeSelected',1,'DelayTimeTXCommandSelected',0,'EncodeSetUnusedBitsToOne',1,'EnableMsgLoopback',0,'TriggerPort',struct('Selected',0,'TriggerType',0),'EnablePortSelected',1,'SignalOnPortnameSelected',1,'UserCoding',struct('Selected',0,'InterfaceFile','UserEncodingFile','FcnName','UserEncodeFcn','InportSelected',0,'InportWidth',1,'OutportSelected',0,'OutportWidth',1),'TerminationMsg',struct('Selected',0,'Byte0_7','0'),'InitialMsg',struct('Selected',0,'Byte0_7','0')),'Message',struct('MsgOnBlocknameSelected',1,'MsgName','EEC1_00','MsgIdFormat',1,'MsgId',217056256,'MsgLength',8,'NumSignals',8,'SampleTime',-1,'StartTime',struct('Selected',0,'Value',0),'AutoRepeatTime',struct('Selected',0,'Value',0.1),'Timeout',struct('Selected',0,'Value',0.1),'DelayTime',struct('Selected',0,'Value',0.1),'Signal',struct('SgnName',{'SPN899_EngineTorqueMode','SPN4154_ActEngPercTorqueFrac','SPN512_DrvrDemEngPercTrq','SPN513_ActEngPercTorque','SPN190_EngineSpeed','SPN1483_SAOfCtrlDevForEngineCtrl','SPN1675_EngineStarterMode','SPN2432_EngDemPercTrq'},'SgnStartBit',{0,4,8,16,24,40,48,56},'SgnLength',{4,4,8,8,16,8,4,8},'SgnType',{0,0,0,0,0,0,0,0},'ModeValue',{-1,-1,-1,-1,-1,-1,-1,-1},'DataType',{0,0,0,0,0,0,0,0},'ByteLayout',{0,0,0,0,0,0,0,0},'Factor',{1,2^-3,1,1,2^-3,1,1,1},'Offset',{0,0,-125,-125,0,0,0,-125},'SgnComment',{{['Engine Torque Mode']},{['Actual Engine - Percent Torque High Resolution']},{['Driver''s Demand Engine - Percent Torque']},{['Actual Engine - Percent Torque']},{['Engine Speed']},{['Source Address of Controlling Device for Engine Control']},{['Engine Starter Mode']},{['Engine Demand – Percent Torque']}},'SgnUnit',{'bit','%','%','%','rpm','SA','bit','%'},'Min',{0,0,-125,-125,0,0,0,-125},'Max',{15,0.875,125,125,8031.875,255,15,125},'SLDataType',{'SS_DOUBLE','SS_DOUBLE','SS_DOUBLE','SS_DOUBLE','SS_DOUBLE','SS_DOUBLE','SS_DOUBLE','SS_DOUBLE'}),'MsgIdNumFormat',1,'MsgComment',{{['Electronic Engine Controller 1']}}),'Version',1.2,'general',struct('isFromLib',0)),'OFF',[]}},'GroupId',{{struct('Group',{{'RTICAN'}},'No',4,'Behavior',{{'NAMECHANGE'}},'BlockType',{{'SINK'}},'NameChangeFlag',0),'OFF',[]}},'SFcnRTICANMessage',{{struct('MsgType','TX','SFcnPortType','Scalar','MsgName','EEC1_00','MsgIdFormat','XTD','MsgId',217056256,'MsgLength',8,'NumSignals',8,'SampleTime',-1,'StartTime',struct('Selected','no','Value',0),'AutoRepeatTime',struct('Selected','no','Value',0.1),'Timeout',struct('Selected','no','Value',0.1),'Signal',struct('SgnName',{'SPN899_EngineTorqueMode','SPN4154_ActEngPercTorqueFrac','SPN512_DrvrDemEngPercTrq','SPN513_ActEngPercTorque','SPN190_EngineSpeed','SPN1483_SAOfCtrlDevForEngineCtrl','SPN1675_EngineStarterMode','SPN2432_EngDemPercTrq'},'SgnStartBit',{0,4,8,16,24,40,48,56},'SgnLength',{4,4,8,8,16,8,4,8},'SgnType',{'standard','standard','standard','standard','standard','standard','standard','standard'},'ModeValue',{-1,-1,-1,-1,-1,-1,-1,-1},'DataType',{['unsigned int'],['unsigned int'],['unsigned int'],['unsigned int'],['unsigned int'],['unsigned int'],['unsigned int'],['unsigned int']},'ByteLayout',{['little endian'],['little endian'],['little endian'],['little endian'],['little endian'],['little endian'],['little endian'],['little endian']},'Factor',{1,2^-3,1,1,2^-3,1,1,1},'Offset',{0,0,-125,-125,0,0,0,-125},'SLDataType',{'SS_DOUBLE','SS_DOUBLE','SS_DOUBLE','SS_DOUBLE','SS_DOUBLE','SS_DOUBLE','SS_DOUBLE','SS_DOUBLE'}),'StatusSelected','yes','TimeSelected','yes','DeltaTimeSelected','yes','DelayTimeSelected','yes','DelayTimeTXCommandSelected','no','EncodeSetUnusedBitsToOne','yes','EnableMsgLoopback','no','TriggerPort',struct('Selected','no','TriggerType',0),'EnablePortSelected','yes','UserCoding',struct('Selected','no','InterfaceFile','UserEncodingFile','FcnName','UserEncodeFcn','InportSelected','no','InportWidth',1,'OutportSelected','no','OutportWidth',1),'TerminationMsg',struct('Selected','no','Byte0','0x00','Byte1','0x00','Byte2','0x00','Byte3','0x00','Byte4','0x00','Byte5','0x00','Byte6','0x00','Byte7','0x00'),'InitialMsg',struct('Selected','no','Byte0','0x00','Byte1','0x00','Byte2','0x00','Byte3','0x00','Byte4','0x00','Byte5','0x00','Byte6','0x00','Byte7','0x00'),'BoardType','DS1','BoardNo',2,'ControllerNo',2),'OFF',[]}},'TLCFileName',{{'rtican_tx_message','OFF',[]}})  RTISFcnParameters=struct('SFcnRTICANMessage','struct','TLCFileName','char')  RTIBlockParaDefault=struct('BoardTypeNo',4302,'BoardNo',1,'ChannelNo',1,'Parameters',struct('DataFileSupport',struct('DataFileSelectedMaster',0,'DataFileSelectedLocal',0,'DataFileName','','DataFileDate','','SelectedFile',['<no file selected>']),'Options',struct('StatusSelected',1,'TimeSelected',1,'DeltaTimeSelected',1,'DelayTimeSelected',1,'DelayTimeTXCommandSelected',0,'EncodeSetUnusedBitsToOne',0,'EnableMsgLoopback',0,'TriggerPort',struct('Selected',0,'TriggerType','rising'),'EnablePortSelected',0,'SignalOnPortnameSelected',1,'UserCoding',struct('Selected',0,'InterfaceFile','UserEncodingFile','FcnName','UserEncodeFcn','InportSelected',0,'InportWidth',1,'OutportSelected',0,'OutportWidth',1),'TerminationMsg',struct('Selected',0,'Byte0_7','0'),'InitialMsg',struct('Selected',0,'Byte0_7','0')),'Message',struct('MsgOnBlocknameSelected',0,'MsgName',['TX Message'],'MsgIdFormat',0,'MsgId',100,'MsgLength',8,'NumSignals',1,'SampleTime',-1,'StartTime',struct('Selected',0,'Value',0),'AutoRepeatTime',struct('Selected',0,'Value',0.1),'Timeout',struct('Selected',0,'Value',0.1),'DelayTime',struct('Selected',0,'Value',0.1),'Signal',struct('SgnName',['TX signal'],'SgnStartBit',0,'SgnLength',8,'SgnType',0,'ModeValue',-1,'DataType',0,'SLDataType','SS_DOUBLE','ByteLayout',0,'Factor',1,'Offset',0,'Min',0,'Max',255,'SgnComment',{{}},'SgnUnit',''),'MsgIdNumFormat',0,'MsgComment',{{''}}),'Version',1.2,'general',struct('isFromLib',1)),'GroupId',struct('Group',{{'RTICAN'}},'No',1,'Behavior',{{'NAMECHANGE'}},'BlockType',{{'SINK'}},'NameChangeFlag',0),'SFcnRTICANMessage',struct('MsgType','TX','MsgName',['TX Message'],'MsgIdFormat','STD','MsgId',100,'MsgLength',2,'NumSignals',1,'SampleTime',-1,'StartTime',struct('Selected','no','Value',0),'AutoRepeatTime',struct('Selected','no','Value',0.1),'Timeout',struct('Selected','no','Value',0.1),'DelayTime',struct('Selected','no','Value',0.1),'Signal',struct('SgnName',['TX signal'],'SgnStartBit',0,'SgnLength',8,'SgnType','standard','ModeValue',-1,'DataType',['unsigned int'],'ByteLayout',['little endian'],'SLDataType','SS_DOUBLE','Factor',1,'Offset',0),'StatusSelected','yes','TimeSelected','yes','DeltaTimeSelected','yes','DelayTimeSelected','yes','EnablePortSelected','no','EnableMsgLoopback','no','DelayTimeTXCommandSelected','no','EncodeSetUnusedBitsToOne','no','UserCoding',struct('Selected','no','InterfaceFile','UserDecodingFile','FcnName','UserDecodeFcn','InportSelected','no','InportWidth',1,'OutportSelected','no','OutportWidth',1),'TerminationMsg',struct('Selected','no','Byte0','0x00','Byte1','0x00','Byte2','0x00','Byte3','0x00','Byte4','0x00','Byte5','0x00','Byte6','0x00','Byte7','0x00'),'InitialMsg',struct('Selected','no','Byte0','0x00','Byte1','0x00','Byte2','0x00','Byte3','0x00','Byte4','0x00','Byte5','0x00','Byte6','0x00','Byte7','0x00'),'TriggerPort',struct('Selected','no','TriggerType','rising'),'BoardType','DS4302','BoardNo',1,'ControllerNo',1,'SFcnPortType','Scalar'),'TLCFileName','rtican_tx_message')
      settings: AttributesFormatString=Group Id: RTICAN4\n  SourceProductName=dSPACE RTI CAN Blockset
  Terminator{,1..3} (4 alike) : Terminator
      settings: InitFcn=|
      | try
      |    MBDS_BlockCallback('Update', gcb);
      | end
  wires:
  Data Type Conversion8/1 -> EEC1_00/8
  Data Type Conversion7/1 -> EEC1_00/7
  Data Type Conversion6/1 -> EEC1_00/6
  Data Type Conversion5/1 -> EEC1_00/5
  Data Type Conversion3/1 -> EEC1_00/4
  Data Type Conversion2/1 -> EEC1_00/3
  Data Type Conversion1/1 -> EEC1_00/2
  Data Type Conversion4/1 -> EEC1_00/1
  Bus Selector/1 -> Data Type Conversion4/1  "<EngTorqueMode>"
  Bus Selector/2 -> Data Type Conversion1/1  "<ActlEngPrcntTrqueHighResolution>"
  Bus Selector/3 -> Data Type Conversion2/1  "<DriversDemandEngPercentTorque>"
  Bus Selector/8 -> Data Type Conversion8/1  "<EngDemandPercentTorque>"
  Bus Selector/4 -> Data Type Conversion3/1  "<ActualEngPercentTorque>"
  Bus Selector/7 -> Data Type Conversion7/1  "<EngStarterMode>"
  Bus Selector/5 -> Data Type Conversion5/1  "<EngSpeed>"
  Bus Selector/6 -> Data Type Conversion6/1  "<SrcAddrssOfCtrllngDvcFrEngCntrl>"
  Data/1 -> Bus Selector/1
  Enable/1 -> EEC1_00/Enable
  EEC1_00/1 -> Terminator/1
  EEC1_00/3 -> Terminator2/1
  EEC1_00/4 -> Terminator3/1
  EEC1_00/2 -> Terminator1/1

== system SUB_ECU_L4_MABX_HW_Interface/CAN_Out_PTC_1571/CAN_TX_10ms/CAN_TX_EEC1_00/TX_CAN5 ==
  Enable : Inport
  Data : Inport  Port=2
  Bus Selector : BusSelector  OutputSignals=INPUTS.CAN.EEC1_00.EngTorqueMode,INPUTS.CAN.EEC1_00.ActlEngPrcntTrqueHighResolution,INPUTS.CAN.EEC1_00.DriversDemandEngPercentTorque,INPUTS.CAN.EEC1_00.ActualEngPercentTorque,INPUTS.CAN.EEC1_00.EngSpeed,INPUTS.CAN.EEC1_00.SrcAddrssOfCtrllngDvcFrEngCntrl,INPUTS.CAN.EEC1_00.EngStarterMode,INPUTS.CAN.EEC1_00.EngDemandPercentTorque
  Data Type Conversion{1..8} (8 alike) : DataTypeConversion  OutDataTypeStr=double  SaturateOnIntegerOverflow=on
  EEC1_00 : rtican/RTICAN Transmit (TX)   Reserved1=[]  Reserved2=[]  Reserved3=[]  Reserved4=[]  SfcnMessage=[]  Msg_Struct=[]  BoardTypeNo=[]  BoardNo=[]  ChannelNo=[]  Parameters=[]  DialogFcn=[]  UnitName=[]  Revision=[]  UnitValues=[]  DSProperties=struct('RTI',struct('Version',uint32(5),'BlockType',struct('isSLSource',uint8(1),'isSLSink',uint8(1),'isHWSource',uint8(0),'isHWSink',uint8(0),'isSetup',uint8(0),'isInline',uint8(1),'isNonInline',uint8(0),'isInterrupt',uint8(0),'isChannelwise',uint8(0)),'IOBoardType','RTICAN','UnitType','MESSAGE','Identifier','TX','DialogType','MSVC','BlockSet','RTICAN','SlaveProcessor','CAN'))  RTIBlockInterface=struct('InputPortsWidth',int32([1 1 1 1 1 1 1 1]),'InputPortsActive',[1 1 1 1 1 1 1 1],'InputPortsName',{{'SPN899_EngineTorqueMode','SPN4154_ActEngPercTorqueFrac','SPN512_DrvrDemEngPercTrq','SPN513_ActEngPercTorque','SPN190_EngineSpeed','SPN1483_SAOfCtrlDevForEngineCtrl','SPN1675_EngineStarterMode','SPN2432_EngDemPercTrq'}},'InputPortsDataType',{{'SS_DOUBLE','SS_DOUBLE','SS_DOUBLE','SS_DOUBLE','SS_DOUBLE','SS_DOUBLE','SS_DOUBLE','SS_DOUBLE'}},'OutputPortsWidth',int32([1 1 1 1]),'OutputPortsActive',[1 1 1 1],'OutputPortsName',{{['TX status'],['TX time'],['TX delta time'],['TX delay time']}},'DialogFcn','rtican_message_interface_gui','BlockDisplay',{{'','center'}},'IconTransparency','on','InitLevel',3,'BlockName',struct('Token',{{'EEC1_00'}}),'SampleTime',{{-1}},'TriggerPort',{{'none'}},'EnablePort',{{'yes'}})  RTIBlockParameters=struct('BoardTypeNo',{{1,'OFF',[]}},'BoardNo',{{3,'ON',[1 16]}},'ChannelNo',{{1,'ON',[1 2]}},'Parameters',{{struct('DataFileSupport',struct('DataFileSelectedMaster',1,'DataFileSelectedLocal',0,'DataFileName','c:\data\svn\truck1571\dbc\mabx_can4_chrisbaltonallstandard.dbc|c:\data\svn\truck1571\dbc\mabx_can4.dbc|','DataFileDate',{{{['16-Jan-2018 13:46:56']}}},'SelectedFile',['<no file selected>']),'Options',struct('StatusSelected',1,'TimeSelected',1,'DeltaTimeSelected',1,'DelayTimeSelected',1,'DelayTimeTXCommandSelected',0,'EncodeSetUnusedBitsToOne',1,'EnableMsgLoopback',0,'TriggerPort',struct('Selected',0,'TriggerType',0),'EnablePortSelected',1,'SignalOnPortnameSelected',1,'UserCoding',struct('Selected',0,'InterfaceFile','UserEncodingFile','FcnName','UserEncodeFcn','InportSelected',0,'InportWidth',1,'OutportSelected',0,'OutportWidth',1),'TerminationMsg',struct('Selected',0,'Byte0_7','0'),'InitialMsg',struct('Selected',0,'Byte0_7','0')),'Message',struct('MsgOnBlocknameSelected',1,'MsgName','EEC1_00','MsgIdFormat',1,'MsgId',217056256,'MsgLength',8,'NumSignals',8,'SampleTime',-1,'StartTime',struct('Selected',0,'Value',0),'AutoRepeatTime',struct('Selected',0,'Value',0.1),'Timeout',struct('Selected',0,'Value',0.1),'DelayTime',struct('Selected',0,'Value',0.1),'Signal',struct('SgnName',{'SPN899_EngineTorqueMode','SPN4154_ActEngPercTorqueFrac','SPN512_DrvrDemEngPercTrq','SPN513_ActEngPercTorque','SPN190_EngineSpeed','SPN1483_SAOfCtrlDevForEngineCtrl','SPN1675_EngineStarterMode','SPN2432_EngDemPercTrq'},'SgnStartBit',{0,4,8,16,24,40,48,56},'SgnLength',{4,4,8,8,16,8,4,8},'SgnType',{0,0,0,0,0,0,0,0},'ModeValue',{-1,-1,-1,-1,-1,-1,-1,-1},'DataType',{0,0,0,0,0,0,0,0},'ByteLayout',{0,0,0,0,0,0,0,0},'Factor',{1,2^-3,1,1,2^-3,1,1,1},'Offset',{0,0,-125,-125,0,0,0,-125},'SgnComment',{{['Engine Torque Mode']},{['Actual Engine - Percent Torque High Resolution']},{['Driver''s Demand Engine - Percent Torque']},{['Actual Engine - Percent Torque']},{['Engine Speed']},{['Source Address of Controlling Device for Engine Control']},{['Engine Starter Mode']},{['Engine Demand – Percent Torque']}},'SgnUnit',{'bit','%','%','%','rpm','SA','bit','%'},'Min',{0,0,-125,-125,0,0,0,-125},'Max',{15,0.875,125,125,8031.875,255,15,125},'SLDataType',{'SS_DOUBLE','SS_DOUBLE','SS_DOUBLE','SS_DOUBLE','SS_DOUBLE','SS_DOUBLE','SS_DOUBLE','SS_DOUBLE'}),'MsgIdNumFormat',1,'MsgComment',{{['Electronic Engine Controller 1']}}),'Version',1.2,'general',struct('isFromLib',0)),'OFF',[]}},'GroupId',{{struct('Group',{{'RTICAN'}},'No',5,'Behavior',{{'NAMECHANGE'}},'BlockType',{{'SINK'}},'NameChangeFlag',0),'OFF',[]}},'SFcnRTICANMessage',{{struct('MsgType','TX','SFcnPortType','Scalar','MsgName','EEC1_00','MsgIdFormat','XTD','MsgId',217056256,'MsgLength',8,'NumSignals',8,'SampleTime',-1,'StartTime',struct('Selected','no','Value',0),'AutoRepeatTime',struct('Selected','no','Value',0.1),'Timeout',struct('Selected','no','Value',0.1),'Signal',struct('SgnName',{'SPN899_EngineTorqueMode','SPN4154_ActEngPercTorqueFrac','SPN512_DrvrDemEngPercTrq','SPN513_ActEngPercTorque','SPN190_EngineSpeed','SPN1483_SAOfCtrlDevForEngineCtrl','SPN1675_EngineStarterMode','SPN2432_EngDemPercTrq'},'SgnStartBit',{0,4,8,16,24,40,48,56},'SgnLength',{4,4,8,8,16,8,4,8},'SgnType',{'standard','standard','standard','standard','standard','standard','standard','standard'},'ModeValue',{-1,-1,-1,-1,-1,-1,-1,-1},'DataType',{['unsigned int'],['unsigned int'],['unsigned int'],['unsigned int'],['unsigned int'],['unsigned int'],['unsigned int'],['unsigned int']},'ByteLayout',{['little endian'],['little endian'],['little endian'],['little endian'],['little endian'],['little endian'],['little endian'],['little endian']},'Factor',{1,2^-3,1,1,2^-3,1,1,1},'Offset',{0,0,-125,-125,0,0,0,-125},'SLDataType',{'SS_DOUBLE','SS_DOUBLE','SS_DOUBLE','SS_DOUBLE','SS_DOUBLE','SS_DOUBLE','SS_DOUBLE','SS_DOUBLE'}),'StatusSelected','yes','TimeSelected','yes','DeltaTimeSelected','yes','DelayTimeSelected','yes','DelayTimeTXCommandSelected','no','EncodeSetUnusedBitsToOne','yes','EnableMsgLoopback','no','TriggerPort',struct('Selected','no','TriggerType',0),'EnablePortSelected','yes','UserCoding',struct('Selected','no','InterfaceFile','UserEncodingFile','FcnName','UserEncodeFcn','InportSelected','no','InportWidth',1,'OutportSelected','no','OutportWidth',1),'TerminationMsg',struct('Selected','no','Byte0','0x00','Byte1','0x00','Byte2','0x00','Byte3','0x00','Byte4','0x00','Byte5','0x00','Byte6','0x00','Byte7','0x00'),'InitialMsg',struct('Selected','no','Byte0','0x00','Byte1','0x00','Byte2','0x00','Byte3','0x00','Byte4','0x00','Byte5','0x00','Byte6','0x00','Byte7','0x00'),'BoardType','DS1','BoardNo',3,'ControllerNo',1),'OFF',[]}},'TLCFileName',{{'rtican_tx_message','OFF',[]}})  RTISFcnParameters=struct('SFcnRTICANMessage','struct','TLCFileName','char')  RTIBlockParaDefault=struct('BoardTypeNo',4302,'BoardNo',1,'ChannelNo',1,'Parameters',struct('DataFileSupport',struct('DataFileSelectedMaster',0,'DataFileSelectedLocal',0,'DataFileName','','DataFileDate','','SelectedFile',['<no file selected>']),'Options',struct('StatusSelected',1,'TimeSelected',1,'DeltaTimeSelected',1,'DelayTimeSelected',1,'DelayTimeTXCommandSelected',0,'EncodeSetUnusedBitsToOne',0,'EnableMsgLoopback',0,'TriggerPort',struct('Selected',0,'TriggerType','rising'),'EnablePortSelected',0,'SignalOnPortnameSelected',1,'UserCoding',struct('Selected',0,'InterfaceFile','UserEncodingFile','FcnName','UserEncodeFcn','InportSelected',0,'InportWidth',1,'OutportSelected',0,'OutportWidth',1),'TerminationMsg',struct('Selected',0,'Byte0_7','0'),'InitialMsg',struct('Selected',0,'Byte0_7','0')),'Message',struct('MsgOnBlocknameSelected',0,'MsgName',['TX Message'],'MsgIdFormat',0,'MsgId',100,'MsgLength',8,'NumSignals',1,'SampleTime',-1,'StartTime',struct('Selected',0,'Value',0),'AutoRepeatTime',struct('Selected',0,'Value',0.1),'Timeout',struct('Selected',0,'Value',0.1),'DelayTime',struct('Selected',0,'Value',0.1),'Signal',struct('SgnName',['TX signal'],'SgnStartBit',0,'SgnLength',8,'SgnType',0,'ModeValue',-1,'DataType',0,'SLDataType','SS_DOUBLE','ByteLayout',0,'Factor',1,'Offset',0,'Min',0,'Max',255,'SgnComment',{{}},'SgnUnit',''),'MsgIdNumFormat',0,'MsgComment',{{''}}),'Version',1.2,'general',struct('isFromLib',1)),'GroupId',struct('Group',{{'RTICAN'}},'No',1,'Behavior',{{'NAMECHANGE'}},'BlockType',{{'SINK'}},'NameChangeFlag',0),'SFcnRTICANMessage',struct('MsgType','TX','MsgName',['TX Message'],'MsgIdFormat','STD','MsgId',100,'MsgLength',2,'NumSignals',1,'SampleTime',-1,'StartTime',struct('Selected','no','Value',0),'AutoRepeatTime',struct('Selected','no','Value',0.1),'Timeout',struct('Selected','no','Value',0.1),'DelayTime',struct('Selected','no','Value',0.1),'Signal',struct('SgnName',['TX signal'],'SgnStartBit',0,'SgnLength',8,'SgnType','standard','ModeValue',-1,'DataType',['unsigned int'],'ByteLayout',['little endian'],'SLDataType','SS_DOUBLE','Factor',1,'Offset',0),'StatusSelected','yes','TimeSelected','yes','DeltaTimeSelected','yes','DelayTimeSelected','yes','EnablePortSelected','no','EnableMsgLoopback','no','DelayTimeTXCommandSelected','no','EncodeSetUnusedBitsToOne','no','UserCoding',struct('Selected','no','InterfaceFile','UserDecodingFile','FcnName','UserDecodeFcn','InportSelected','no','InportWidth',1,'OutportSelected','no','OutportWidth',1),'TerminationMsg',struct('Selected','no','Byte0','0x00','Byte1','0x00','Byte2','0x00','Byte3','0x00','Byte4','0x00','Byte5','0x00','Byte6','0x00','Byte7','0x00'),'InitialMsg',struct('Selected','no','Byte0','0x00','Byte1','0x00','Byte2','0x00','Byte3','0x00','Byte4','0x00','Byte5','0x00','Byte6','0x00','Byte7','0x00'),'TriggerPort',struct('Selected','no','TriggerType','rising'),'BoardType','DS4302','BoardNo',1,'ControllerNo',1,'SFcnPortType','Scalar'),'TLCFileName','rtican_tx_message')
      settings: AttributesFormatString=Group Id: RTICAN5\n  SourceProductName=dSPACE RTI CAN Blockset
  Terminator{,1..3} (4 alike) : Terminator
      settings: InitFcn=|
      | try
      |    MBDS_BlockCallback('Update', gcb);
      | end
  wires:
  EEC1_00/2 -> Terminator1/1
  EEC1_00/4 -> Terminator3/1
  EEC1_00/3 -> Terminator2/1
  EEC1_00/1 -> Terminator/1
  Enable/1 -> EEC1_00/Enable
  Data/1 -> Bus Selector/1
  Bus Selector/6 -> Data Type Conversion6/1  "<SrcAddrssOfCtrllngDvcFrEngCntrl>"
  Bus Selector/5 -> Data Type Conversion5/1  "<EngSpeed>"
  Bus Selector/7 -> Data Type Conversion7/1  "<EngStarterMode>"
  Bus Selector/4 -> Data Type Conversion3/1  "<ActualEngPercentTorque>"
  Bus Selector/8 -> Data Type Conversion8/1  "<EngDemandPercentTorque>"
  Bus Selector/3 -> Data Type Conversion2/1  "<DriversDemandEngPercentTorque>"
  Bus Selector/2 -> Data Type Conversion1/1  "<ActlEngPrcntTrqueHighResolution>"
  Bus Selector/1 -> Data Type Conversion4/1  "<EngTorqueMode>"
  Data Type Conversion4/1 -> EEC1_00/1
  Data Type Conversion1/1 -> EEC1_00/2
  Data Type Conversion2/1 -> EEC1_00/3
  Data Type Conversion3/1 -> EEC1_00/4
  Data Type Conversion5/1 -> EEC1_00/5
  Data Type Conversion6/1 -> EEC1_00/6
  Data Type Conversion7/1 -> EEC1_00/7
  Data Type Conversion8/1 -> EEC1_00/8
